simulink model "lab4_model_2"  (R2015a)
settings: Solver=ode45  StartTime=0.0  StopTime=10.0  RelTol=1e-3
settings Model: Creator=bb  LastModifiedBy=bb

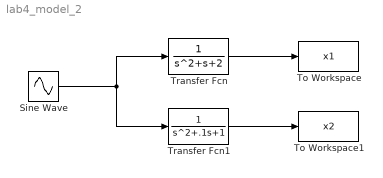
== system lab4_model_2 ==
  Sine Wave : Sin  SampleTime=0
  To Workspace : ToWorkspace  VariableName=x1  SaveFormat=Timeseries  SampleTime=-1
  To Workspace1 : ToWorkspace  VariableName=x2  SaveFormat=Timeseries  SampleTime=-1
  Transfer Fcn : TransferFcn  Denominator=[1 1 2]
  Transfer Fcn1 : TransferFcn  Denominator=[1 .1 1]
  wires:
  Sine Wave/1 -> Transfer Fcn1/1, Transfer Fcn/1
  Transfer Fcn/1 -> To Workspace/1
  Transfer Fcn1/1 -> To Workspace1/1
